simulink model "notcontroledsystem"  (R2014b)
settings: Solver=VariableStepAuto  StartTime=0.0  StopTime=20  RelTol=1e-3
libraries: simulink x1
settings Model: Creator=ASUS  LastModifiedBy=Signal
settings DataIOCC: LimitDataPoints=off  SaveFormat=Dataset
settings OptimizationCC: UseDivisionForNetSlopeComputation=off  LifeSpan=auto  SimCompilerOptimization=off
settings DebuggingCC: SolverPrmCheckMsg=none  FcnCallInpInsideContextMsg=error  FrameProcessingCompatibilityMsg=error  LibraryContextMissingDiagnostic=warning  SFUnexpectedBacktrackingDiag=error  SFNoUnconditionalDefaultTransitionDiag=error
settings HardwareCC: ProdBitPerPointer=64  ProdLargestAtomicFloat=Float  ProdIntDivRoundTo=Zero  ProdEndianess=LittleEndian  ProdWordSize=64  ProdHWDeviceType=Intel->x86-64 (Windows64)
settings ModelReferenceCC: PropagateSignalLabelsOutOfModel=on
settings SFSimCC: SimUseLocalCustomCode=on
settings RTWCC: RTWUseLocalCustomCode=on  RTWCompilerOptimization=off
settings GRTTargetCC: TargetLangStandard=C99 (ISO)  GeneratePreprocessorConditionals=Use local settings

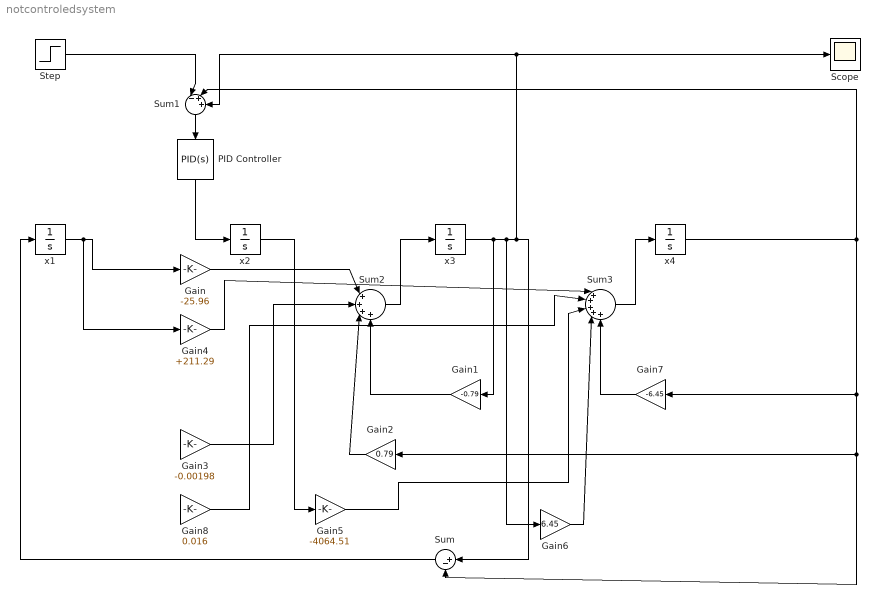
== system notcontroledsystem ==
  Gain : Gain  Gain=-25.96
  Gain1 : Gain  Gain=-0.79
  Gain2 : Gain  Gain=0.79
  Gain3 : Gain  Gain=-0.00198
  Gain4 : Gain  Gain=+211.29
  Gain5 : Gain  Gain=-4064.51
  Gain6 : Gain  Gain=6.45
  Gain7 : Gain  Gain=-6.45
  Gain8 : Gain  Gain=0.016
  PID Controller : simulink/Continuous/PID Controller  Controller=PID  TimeDomain=Continuous-time  SampleTime=-1  IntegratorMethod=Forward Euler  FilterMethod=Forward Euler  Form=Parallel  P=800  I=3500  D=5000  N=100  InitialConditionSource=internal  InitialConditionForIntegrator=0  InitialConditionForFilter=0  ExternalReset=none  LimitOutput=off  UpperSaturationLimit=inf  LowerSaturationLimit=-inf  LinearizeAsGain=on  AntiWindupMode=none  Kb=1  TrackingMode=off  Kt=1  PParamMin=[]  PParamMax=[]  IParamMin=[]  IParamMax=[]  DParamMin=[]  DParamMax=[]  NParamMin=[]  NParamMax=[]  KbParamMin=[]  KbParamMax=[]  KtParamMin=[]  KtParamMax=[]  POutMin=[]  POutMax=[]  IOutMin=[]  IOutMax=[]  DOutMin=[]  DOutMax=[]  NOutMin=[]  NOutMax=[]  KbOutMin=[]  KbOutMax=[]  KtOutMin=[]  KtOutMax=[]  IntegratorOutMin=[]  IntegratorOutMax=[]  FilterOutMin=[]  FilterOutMax=[]  SumOutMin=[]  SumOutMax=[]  SumI1OutMin=[]  SumI1OutMax=[]  SumI2OutMin=[]  SumI2OutMax=[]  SumI3OutMin=[]  SumI3OutMax=[]  SumDOutMin=[]  SumDOutMax=[]  SaturationOutMin=[]  SaturationOutMax=[]  IntegratorContinuousStateAttributes=''  IntegratorStateMustResolveToSignalObject=off  IntegratorRTWStateStorageClass=Auto  FilterContinuousStateAttributes=''  FilterStateMustResolveToSignalObject=off  FilterRTWStateStorageClass=Auto  DifferentiatorICPrevScaledInput=0  DifferentiatorOutMin=[]  DifferentiatorOutMax=[]  UseFilter=on
  Scope : Scope
      settings: YMin=-0.00039  YMax=0.00032
  Step : Step  SampleTime=0
  Sum : Sum  Inputs=|+-
  Sum1 : Sum  Inputs=|-++
  Sum2 : Sum  Inputs=|++++
  Sum3 : Sum  Inputs=|+++++
  x{1..4} (4 alike) : Integrator
  wires:
  Sum/1 -> x1/1
  x1/1 -> Gain4/1, Gain/1
  x2/1 -> Gain5/1
  Sum3/1 -> x4/1
  x4/1 -> Sum1/2, Gain7/1, Gain2/1, Sum/2
  Sum2/1 -> x3/1
  Step/1 -> Sum1/1
  Gain/1 -> Sum2/1
  Gain3/1 -> Sum2/2
  Gain2/1 -> Sum2/3
  Gain1/1 -> Sum2/4
  Gain4/1 -> Sum3/1
  Gain8/1 -> Sum3/2
  Gain5/1 -> Sum3/3
  Gain6/1 -> Sum3/4
  Gain7/1 -> Sum3/5
  ? -> Gain8/1, Gain3/1
  x3/1 -> Gain1/1, Gain6/1, Scope/1, Sum1/3, Sum/1
  Sum1/1 -> PID Controller/1
  PID Controller/1 -> x2/1
